simulink model "untitled1"  (R2020a)
settings: Solver=FixedStepAuto  StartTime=0.0  StopTime=40  FixedStep=0.001  RelTol=1e-3
values from neighbouring files (symbols this model uses):
  K = getBlockValue(T, 'k')    [Copy_of_init_hinf.m]    (also in init_hinf.m; init_lqr.m = lqr(G.A, -G.B, Q, R))
undefined symbols (not defined in the file or in its folder): sigbuilder_block
settings Model: Creator=dvieira  LastModifiedBy=dvieira

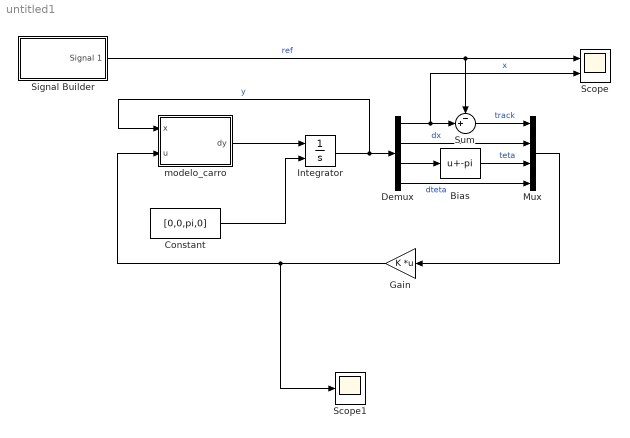
== system untitled1 ==
  Bias : Bias  Bias=-pi
  Constant : Constant  Value=[0,0,pi,0]
  Demux : Demux
  Gain : Gain  Gain=K  Multiplication=Matrix(K*u)
  Integrator : Integrator  InitialConditionSource=external  InitialCondition=[1]
  Mux : Mux
  Scope : Scope  NumInputPorts=2
  Scope1 : Scope
  Signal Builder : Subsystem  Tag=STV Subsys  LoadFcn=sigbuilder_block('load');  StartFcn=sigbuilder_block('start');  StopFcn=sigbuilder_block('stop');  ClipboardFcn=sigbuilder_block('clipboard');  mask(Sigbuilder block){tuvar=[0:10]}
      mask help: Simulink:masks:SigbuilderBlock_MD
      mask init:
      | if ~strcmp(get_param(bdroot(gcbh),'SimulationStatus'),'stopped') tuvar = sigbuilder_block('maskInit'); end
      settings: CopyFcn=sigbuilder_block('copy');  DeleteFcn=sigbuilder_block('delete');  ModelCloseFcn=sigbuilder_block('modelClose');  PreSaveFcn=sigbuilder_block('preSave');  PauseFcn=sigbuilder_block('pause');  ContinueFcn=sigbuilder_block('continue');  NameChangeFcn=sigbuilder_block('namechange');  OpenFcn=sigbuilder_block('open',[233.25 157.5 550.5 399.75 ]);  CloseFcn=sigbuilder_block('close');
      mask Display: plot(0, 0, 100, 100,[2, 2, 32, 32, 2], [68, 8, 8, 68, 68],[32, 2], [38, 38], [32, 19, 2],[53, 60, 44], [32, 17, 17, 2],[16, 16, 31, 31]);txt = getActiveGroup(gcbh);text(2, 100, txt,'verticalAlignment', 'top');
  Sum : Sum  Inputs=-+|
  modelo_carro : MATLAB Function  TreatAsAtomicUnit=on
  wires:
  Gain/1 -> Scope1/1, modelo_carro/2(u)
  modelo_carro/1(dy) -> Integrator/1
  Signal Builder/1(Signal 1) -> Scope/1, Sum/1  "ref"
  Demux/1 -> Scope/2, Sum/2  "x"
  Sum/1 -> Mux/1  "track"
  Demux/2 -> Mux/2  "dx"
  Demux/3 -> Bias/1
  Demux/4 -> Mux/4  "dteta"
  Mux/1 -> Gain/1
  Integrator/1 -> modelo_carro/1(x), Demux/1  "y"
  Constant/1 -> Integrator/2
  Bias/1 -> Mux/3  "teta"

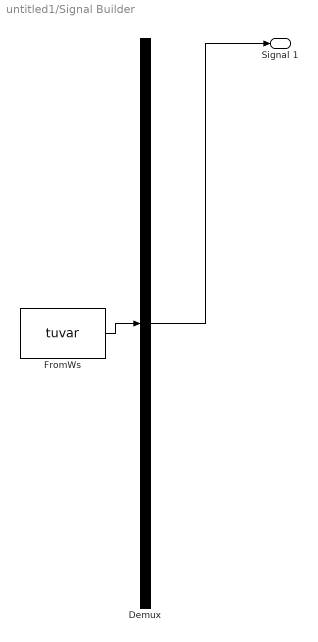
== system untitled1/Signal Builder ==
  Demux : Demux  Tag=STV Demux  Outputs=1
      settings: DisplayOption=none
  FromWs : FromWorkspace  Tag=STV FromWs  VariableName=tuvar
      SigBuilderData=|
      | common.afterFinalStr = 'Extrapolate'
      | common.sampleTime = 0
      | dataSet.timeRange = [0 40]
      | dataSet.name = 'Group 1'
      | sbobj.Groups.Name = 'Group 1'
      | sbobj.Groups.Signals.Name = 'Signal 1'
      | sbobj.Groups.Signals.XData = [0 4 4 14 14 21.8 27.8 27.8 32.6 32.6 40]
      | sbobj.Groups.Signals.YData = [0 0 1 1 3 3 1.6 1.1 1.1 0 0]
      | sbobj.Groups.TimeRange = [0 40]
  Signal 1 : Outport  Tag=STV Outport
  wires:
  Demux/1 -> Signal 1/1
  FromWs/1 -> Demux/1

== matlab function untitled1/modelo_carro ==
  data: x input; u input; dy output
function dy = fcn(x,u)
    m = 1.0;
    M = 5.0;
    L = 2.0;
    g = -10.0;
    d = 1.0;
    dy = fn_eq_diferencial(x,m,M,L,g,d,u);
